simulink model "EV_thermal_charger_2015a_20200311"  (R2015a)
settings: Solver=ode3  StartTime=0.0  StopTime=1800  FixedStep=sampling_time  RelTol=1e-3
PreLoadFcn:
  | run('init_setting.m')
PostLoadFcn:
  | set_param(gcs, 'SimulationCommand', 'update');
  | load('save_param/save_P_Charger', 'P_Charger');
  | load('save_param/save_T_User_set_temp_degC','T_User_set_temp_degC');
  | load('save_param/save_ENV_PNT_PTTH_Temp_add_degC','ENV_PNT_PTTH_Temp_add_degC');
  | load('save_param/save_ENV_PNT_CABIN_Temp_add_degC','ENV_PNT_CABIN_Temp_add_degC');
  | load('save_param/save_ENV_PNT_PHI_Sunlight_W','ENV_PNT_PHI_Sunlight_W');
  | load('save_param/save_ENV_PNT_Outside_Temp_ini_degC','ENV_PNT_Outside_Temp_ini_degC');
undefined symbols (not defined in the file or in its folder): BK_PNT_Pow_UL, BK_PNT_ReGene_vel_limit_DN_kmph, BK_PNT_ReGene_vel_limit_UP_kmph, BK_PNT_Tau_brake, Brk_LL, Brk_PGain, Brk_UL, BT_PNT_Hi_C_pol_hi_batt, BT_PNT_Hi_Capa_hi_batt_F, BT_PNT_Hi_ocv_SOC_hi_batt_OCV_V_table, BT_PNT_Hi_ocv_SOC_hi_batt_OCV_V_table_x_SOC, BT_PNT_Hi_R_hi_batt_cell, BT_PNT_Hi_R_pol_hi_batt, BT_PNT_Hi_SOC_MAX_hi_batt, BT_PNT_Hi_SOC_MIN_hi_batt, BT_PNT_Hi_SOC_START_hi_batt, BT_PNT_Lo_Capa_lo_batt_F, BT_PNT_Lo_ocv_SOC_lo_batt_OCV_V_table, BT_PNT_Lo_ocv_SOC_lo_batt_OCV_V_table_x_SOC, BT_PNT_Lo_R_lo_batt_ohm, BT_PNT_Lo_SOC_MAX_lo_batt, BT_PNT_Lo_SOC_MIN_lo_batt, BT_PNT_Lo_SOC_START_lo_batt, BTTH_CNT_P_BT_Heater_W, BTTH_CNT_P_BT_Heater_W_x_BTCells_degC, BTTH_CNT_Voltage_BTFan_V, BTTH_CNT_Voltage_BTFan_V_x_BTCells_degC, BTTH_PNT_BT_Heat_Resi_KpW, BTTH_PNT_BT_Heat_Resi_KpW_x_Wind_m3ps, BTTH_PNT_BT_Heater2BTCells_Heat_Resi_KpW, BTTH_PNT_BT_Heater_Heat_Capa_JpK, BTTH_PNT_BTBlock2BTAir_Heat_Resi_KpW, BTTH_PNT_BTBlock_Heat_Capa_JpK, BTTH_PNT_BTCells2BTBlock_Heat_Resi_KpW, BTTH_PNT_BTCells_Heat_Capa_JpK, BTTH_PNT_v_BTFan_Wind_vel_mps, BTTH_PNT_v_BTFan_Wind_vel_mps_x_V_BTFan, CATH_CNT_P_Aircon_W_LL, CATH_CNT_P_Aircon_W_UL, CATH_CNT_P_Gain_Aircon, CATH_CNT_P_Gain_PTC_Heater, CATH_CNT_P_Gain_SeatHT, CATH_CNT_P_PTC_Heater, CATH_CNT_P_PTC_Heater_W_LL, CATH_CNT_P_PTC_Heater_W_UL, CATH_CNT_P_PTC_Heater_x_T_Outside_temp_degC, CATH_CNT_P_SeatHT_W_LL, CATH_CNT_P_SeatHT_W_UL, CATH_CNT_PGain_Temp_blowout, CATH_CNT_T_Aircon_Indoor_degC, CATH_CNT_T_Aircon_Indoor_degC_x_T_blowout_degC, CATH_CNT_T_PTC_Heater_degC_UL, CATH_CNT_T_SeatHT_Temp_degC, CATH_CNT_T_SeatHT_Temp_degC_x_T_blowout_degC, CATH_CNT_V_HVAC_Fan, CATH_CNT_V_HVAC_Fan_x_T_blowout_degC, CATH_CNT_V_RDFan_V, CATH_CNT_V_RDFan_x_P_Aircon_W, CATH_PNT_Air_Convection_Heat_Resi_KpW, CATH_PNT_Air_Convection_Heat_Resi_x_mps ... (+141)
undefined symbols (not defined in the file): ACC_D_Gain, ACC_I_Gain, ACC_P_Gain
libraries: METI_Lib_vehicle_model x52, simulink x35
(part 3 of 6)

== system EV_thermal_charger_2015a_20200311/Vehicle/BT_Hi_PNT/Subsystem ==
  I_BT_PNT_A : Inport
  Add : Sum
  Divide : Product
  Resistivity : Constant  Value=BT_PNT_Hi_R_hi_batt_cell
  Transfer Fcn : TransferFcn  Numerator=[BT_PNT_Hi_R_pol_hi_batt]  Denominator=[BT_PNT_Hi_R_pol_hi_batt*BT_PNT_Hi_C_pol_hi_batt 1]
  V_BT_PNT_V : Outport
  wires:
  Resistivity/1 -> Divide/2
  I_BT_PNT_A/1 -> Transfer Fcn/1, Divide/1
  Divide/1 -> Add/1
  Transfer Fcn/1 -> Add/2
  Add/1 -> V_BT_PNT_V/1

== system EV_thermal_charger_2015a_20200311/Vehicle/BT_Lo_PNT/Cal_SOC ==
  I_Lo_BT_PNT_A : Inport
  Capa_batt : Inport  Port=2
  SOC_st : Inport  Port=3
  SOC_MAX : Inport  Port=4
  SOC_MIN : Inport  Port=5
  Clock : Clock
  Memory : Memory
  Memory1 : Memory
  Saturation Dynamic : simulink/Discontinuities/Saturation Dynamic  OutMin=[]  OutMax=[]  OutDataTypeStr=Inherit: Same as second input  OutDataType=fixdt(1, 16)  OutScaling=2^-10  DoSatur=off
  Sum : Sum  Inputs=|++
  Sum1 : Sum  Inputs=++|
  Sum2 : Sum  Inputs=+-|
  Sum5 : Sum  Inputs=|+-
  capa_mn : Product  RndMeth=Zero
  capa_mx : Product  RndMeth=Zero
  capa_mx1 : Product  RndMeth=Zero
  capa_st : Product  RndMeth=Zero
  capa_st1 : Product  Inputs=*/  RndMeth=Zero
  h2sec : Gain  Gain=h2sec
  k : Gain  Gain=percent2mujigen
  k1 : Gain  Gain=percent2mujigen
  k2 : Gain  Gain=percent2mujigen
  k3 : Gain  Gain=mujigen2percent
  SOC_out : Outport
  wires:
  Sum5/1 -> capa_mx1/2
  Memory1/1 -> Sum5/2
  Sum/1 -> Saturation Dynamic/2
  Clock/1 -> Sum5/1, Memory1/1
  capa_mx1/1 -> Sum1/1
  k3/1 -> SOC_out/1
  Sum1/1 -> Sum/2
  Memory/1 -> Sum1/2
  k2/1 -> capa_st/2
  k1/1 -> capa_mn/2
  k/1 -> capa_mx/2
  capa_st/1 -> Sum2/2, Sum/1
  Saturation Dynamic/1 -> Sum2/1, capa_st1/1
  capa_mx/1 -> Saturation Dynamic/1
  capa_mn/1 -> Saturation Dynamic/3
  capa_st1/1 -> k3/1
  h2sec/1 -> capa_mn/1, capa_st1/2, capa_st/1, capa_mx/1
  SOC_MIN/1 -> k1/1
  SOC_MAX/1 -> k/1
  SOC_st/1 -> k2/1
  Capa_batt/1 -> h2sec/1
  I_Lo_BT_PNT_A/1 -> capa_mx1/1
  Sum2/1 -> Memory/1

== system EV_thermal_charger_2015a_20200311/Vehicle/BT_Lo_PNT/Subsystem ==
  I_BT_PNT_Lo_A : Inport
  Divide : Product
  Resistivity : Constant  Value=BT_PNT_Lo_R_lo_batt_ohm
  V_BT_PNT_Lo_V : Outport
  wires:
  Resistivity/1 -> Divide/2
  I_BT_PNT_Lo_A/1 -> Divide/1
  Divide/1 -> V_BT_PNT_Lo_V/1

== system EV_thermal_charger_2015a_20200311/Vehicle/CATH_CNT/Calc_Temp_Blowout ==
  tSetting_T_User_set_temp_degC : Inport
  T_ATM_PNT_Outside_degC : Inport  Port=2
  T_CABA_PNT_T : Inport  Port=3
  v_vehicle_mps_1 : Inport  Port=4
  Add : Sum
  Constant : Constant  Value=CATH_PNT_CABIN_AIR_Heat_Capa_JpK
  Divide : Product  Inputs=*/
  FB : Subsystem
  FF1 : Subsystem
  Gain : Gain  Gain=0.05
  Subtract : Sum  Inputs=-+
  Subtract1 : Sum  Inputs=+-
  T_blowout_degC : Outport
  T_diff_temp_degC : Outport  Port=2
  wires:
  T_CABA_PNT_T/1 -> FF1/2(T_CABIN_AIR_temp_degC), Subtract/2
  T_ATM_PNT_Outside_degC/1 -> FF1/1(T_Outside_temp_degC)
  Add/1 -> Divide/1
  Divide/1 -> Subtract1/2, T_blowout_degC/1
  Constant/1 -> Gain/1
  Subtract/1 -> Subtract1/1, FB/1(T_diff_temp_degC)
  tSetting_T_User_set_temp_degC/1 -> Subtract/1
  Subtract1/1 -> T_diff_temp_degC/1
  FB/1(Q_FB) -> Add/1
  Gain/1 -> Divide/2
  v_vehicle_mps_1/1 -> FF1/3(v_vehicle_mps)
  FF1/1(Q_Heat_Transfar) -> Add/2

== system EV_thermal_charger_2015a_20200311/Vehicle/CATH_CNT/P_Heatpomp_Power_tgt_calc ==
  note: A/CフラグがON かつ Auto Wind ONの時はヒートポンプ稼働
  T_diff_temp_degC : Inport
  T_AC_PNT_Indoor_degC : Inport  Port=2
  Flag_Aircon : Inport  Port=3
  Flag_AutoWind : Inport  Port=4
  Abs : Abs
  Compare To Constant : simulink/Logic and Bit Operations/Compare To Constant  relop=>  const=0.5  OutDataTypeStr=boolean
  Compare To Constant1 : simulink/Logic and Bit Operations/Compare To Constant  relop=>  const=0.5  OutDataTypeStr=boolean
  Constant : Constant  Value=CATH_CNT_P_Gain_Aircon
  Constant1 : Constant  Value=CATH_CNT_P_Aircon_W_UL
  Constant2 : Constant  Value=CATH_CNT_P_Aircon_W_LL
  Constant3 : Constant  Value=0
  Gain1 : Gain  Gain=-1
  Logical Operator : Logic  AllPortsSameDT=off  OutDataTypeStr=boolean
  Product : Product
  Saturation Dynamic : simulink/Discontinuities/Saturation Dynamic  OutMin=[]  OutMax=[]  OutDataTypeStr=Inherit: Same as second input  OutDataType=fixdt(1, 16)  OutScaling=2^-10  DoSatur=off
  Subtract : Sum
  Switch : Switch  Criteria=u2 > Threshold
  T_Aircon_Indoor_tgt : Lookup_n-D  NumberOfTableDimensions=1  BreakpointsForDimension1=CATH_CNT_T_Aircon_Indoor_degC_x_T_blowout_degC  BeginIndexSearchUsingPreviousIndexResult=on  Table=CATH_CNT_T_Aircon_Indoor_degC  ExtrapMethod=Clip  InternalRulePriority=Speed  RndMeth=Simplest  InputSameDT=on
  V_RDFan_tgt1 : Lookup_n-D  NumberOfTableDimensions=1  BreakpointsForDimension1=CATH_CNT_V_RDFan_x_P_Aircon_W  BeginIndexSearchUsingPreviousIndexResult=on  Table=CATH_CNT_V_RDFan_V  ExtrapMethod=Clip  UseLastTableValue=on  InternalRulePriority=Speed  RndMeth=Simplest  InputSameDT=on
  P_CATH_CNT_Heatpomp_W : Outport
  req_V_CATH_CNT_RDFan_V : Outport  Port=2
  wires:
  T_diff_temp_degC/1 -> T_Aircon_Indoor_tgt/1
  T_Aircon_Indoor_tgt/1 -> Subtract/1
  T_AC_PNT_Indoor_degC/1 -> Gain1/1
  Subtract/1 -> Product/1
  Constant/1 -> Product/2
  Product/1 -> Saturation Dynamic/2
  Constant1/1 -> Saturation Dynamic/1
  Constant2/1 -> Saturation Dynamic/3
  Flag_Aircon/1 -> Compare To Constant/1
  Saturation Dynamic/1 -> Switch/1
  Logical Operator/1 -> Switch/2
  Constant3/1 -> Switch/3
  Switch/1 -> Abs/1, P_CATH_CNT_Heatpomp_W/1
  V_RDFan_tgt1/1 -> req_V_CATH_CNT_RDFan_V/1
  Flag_AutoWind/1 -> Compare To Constant1/1
  Compare To Constant/1 -> Logical Operator/1
  Compare To Constant1/1 -> Logical Operator/2
  Gain1/1 -> Subtract/2
  Abs/1 -> V_RDFan_tgt1/1

== system EV_thermal_charger_2015a_20200311/Vehicle/CATH_CNT/P_PTC_Heater_tgt_calc ==
  note: エアコンフラグがONの時は
      | PTCヒーターは使用しない
  note: ヒーター温度が上限値を超過した場合に
      | ヒーター出力を下げる制御
  note: A/CフラグがOFF かつ Auto Wind ONの時
      | PTCヒーターを使用
  T_ATM_PNT_Outside_degC : Inport
  T_PTC_PNT_degC : Inport  Port=2
  Flag_Aircon : Inport  Port=3
  Flag_AutoWind : Inport  Port=4
  Add : Sum
  Compare To Constant : simulink/Logic and Bit Operations/Compare To Constant  relop=>  const=0.5  OutDataTypeStr=boolean
  Compare To Constant1 : simulink/Logic and Bit Operations/Compare To Constant  relop=>  const=0.5  OutDataTypeStr=boolean
  Constant : Constant  Value=CATH_CNT_P_Gain_PTC_Heater
  Constant1 : Constant  Value=CATH_CNT_P_PTC_Heater_W_UL
  Constant2 : Constant  Value=CATH_CNT_P_PTC_Heater_W_LL
  Constant3 : Constant  Value=CATH_CNT_T_PTC_Heater_degC_UL
  Constant4 : Constant  Value=0
  Constant5 : Constant  Value=-inf
  Constant6 : Constant  Value=0
  Logical Operator : Logic  Operator=NOT  AllPortsSameDT=off  OutDataTypeStr=boolean
  Logical Operator1 : Logic  AllPortsSameDT=off  OutDataTypeStr=boolean
  P_PTC_Heater_tgt : Lookup_n-D  NumberOfTableDimensions=1  BreakpointsForDimension1=CATH_CNT_P_PTC_Heater_x_T_Outside_temp_degC  BeginIndexSearchUsingPreviousIndexResult=on  Table=CATH_CNT_P_PTC_Heater  ExtrapMethod=Clip  InternalRulePriority=Speed  RndMeth=Simplest  InputSameDT=on
  Product : Product
  Saturation Dynamic : simulink/Discontinuities/Saturation Dynamic  OutMin=[]  OutMax=[]  OutDataTypeStr=Inherit: Same as second input  OutDataType=fixdt(1, 16)  OutScaling=2^-10  DoSatur=off
  Saturation Dynamic1 : simulink/Discontinuities/Saturation Dynamic  OutMin=[]  OutMax=[]  OutDataTypeStr=Inherit: Same as second input  OutDataType=fixdt(1, 16)  OutScaling=2^-10  DoSatur=off
  Subtract : Sum  Inputs=+-
  Switch : Switch  Criteria=u2 > Threshold
  P_CATH_CNT_PTC_Heater_W : Outport
  wires:
  T_ATM_PNT_Outside_degC/1 -> P_PTC_Heater_tgt/1
  Subtract/1 -> Saturation Dynamic1/2
  Constant/1 -> Product/2
  Add/1 -> Saturation Dynamic/2
  Constant1/1 -> Saturation Dynamic/1
  Constant2/1 -> Saturation Dynamic/3
  T_PTC_PNT_degC/1 -> Subtract/2
  Saturation Dynamic/1 -> Switch/1
  Constant3/1 -> Subtract/1
  Saturation Dynamic1/1 -> Product/1
  Constant4/1 -> Saturation Dynamic1/1
  Constant5/1 -> Saturation Dynamic1/3
  P_PTC_Heater_tgt/1 -> Add/1
  Product/1 -> Add/2
  Flag_Aircon/1 -> Compare To Constant/1
  Compare To Constant/1 -> Logical Operator/1
  Constant6/1 -> Switch/3
  Switch/1 -> P_CATH_CNT_PTC_Heater_W/1
  Logical Operator1/1 -> Switch/2
  Compare To Constant1/1 -> Logical Operator1/2
  Flag_AutoWind/1 -> Compare To Constant1/1
  Logical Operator/1 -> Logical Operator1/1

== system EV_thermal_charger_2015a_20200311/Vehicle/CATH_CNT/Subsystem1 ==
  tSetting_P_Charger : Inport
  Compare To Zero : simulink/Logic and Bit Operations/Compare To Zero  relop=>  OutDataTypeStr=boolean
  Constant1 : Constant
  Constant3 : Constant  Value=0
  Switch : Switch  Criteria=u2 > Threshold
  Switch1 : Switch  Criteria=u2 > Threshold
  Flag_Aircon : Outport
  Flag_AutoWind : Outport  Port=2
  wires:
  Switch/1 -> Flag_Aircon/1
  Switch1/1 -> Flag_AutoWind/1
  Compare To Zero/1 -> Switch1/2, Switch/2
  tSetting_P_Charger/1 -> Compare To Zero/1
  Constant3/1 -> Switch1/1, Switch/1
  Constant1/1 -> Switch1/3, Switch/3

== system EV_thermal_charger_2015a_20200311/Vehicle/CATH_CNT/T_SeatHT_Temp_tgt_calc ==
  T_diff_temp_degC : Inport
  T_SH_PNT_degC : Inport  Port=2
  Constant : Constant  Value=CATH_CNT_P_Gain_SeatHT
  Constant1 : Constant  Value=CATH_CNT_P_SeatHT_W_UL
  Constant2 : Constant  Value=CATH_CNT_P_SeatHT_W_LL
  Product : Product
  Saturation Dynamic : simulink/Discontinuities/Saturation Dynamic  OutMin=[]  OutMax=[]  OutDataTypeStr=Inherit: Same as second input  OutDataType=fixdt(1, 16)  OutScaling=2^-10  DoSatur=off
  Subtract : Sum  Inputs=+-
  T_SeatHT_Temp_tgt : Lookup_n-D  NumberOfTableDimensions=1  BreakpointsForDimension1=CATH_CNT_T_SeatHT_Temp_degC_x_T_blowout_degC  BeginIndexSearchUsingPreviousIndexResult=on  Table=CATH_CNT_T_SeatHT_Temp_degC  ExtrapMethod=Clip  InternalRulePriority=Speed  RndMeth=Simplest  InputSameDT=on
  P_CATH_CNT_SeatHT_W : Outport
  wires:
  T_diff_temp_degC/1 -> T_SeatHT_Temp_tgt/1
  Subtract/1 -> Product/1
  Constant/1 -> Product/2
  Product/1 -> Saturation Dynamic/2
  Constant1/1 -> Saturation Dynamic/1
  Constant2/1 -> Saturation Dynamic/3
  T_SeatHT_Temp_tgt/1 -> Subtract/1
  T_SH_PNT_degC/1 -> Subtract/2
  Saturation Dynamic/1 -> P_CATH_CNT_SeatHT_W/1

== system EV_thermal_charger_2015a_20200311/Vehicle/CATH_CNT/V_HVAC_Fan_calc ==
  T_diff_temp_degC : Inport
  Flag_AutoWind_ON : Inport  Port=2
  Compare To Constant1 : simulink/Logic and Bit Operations/Compare To Constant  relop=>  const=0.5  OutDataTypeStr=boolean
  Constant : Constant  Value=0
  Switch : Switch  Criteria=u2 > Threshold  Threshold=0.5
  V_HVAC_Fan : Lookup_n-D  NumberOfTableDimensions=1  BreakpointsForDimension1=CATH_CNT_V_HVAC_Fan_x_T_blowout_degC  BeginIndexSearchUsingPreviousIndexResult=on  Table=CATH_CNT_V_HVAC_Fan  ExtrapMethod=Clip  InternalRulePriority=Speed  RndMeth=Simplest  InputSameDT=on
  V_CATH_CNT_Aircon_Fan_V : Outport
  wires:
  T_diff_temp_degC/1 -> V_HVAC_Fan/1
  V_HVAC_Fan/1 -> Switch/1
  Flag_AutoWind_ON/1 -> Compare To Constant1/1
  Constant/1 -> Switch/3
  Switch/1 -> V_CATH_CNT_Aircon_Fan_V/1
  Compare To Constant1/1 -> Switch/2

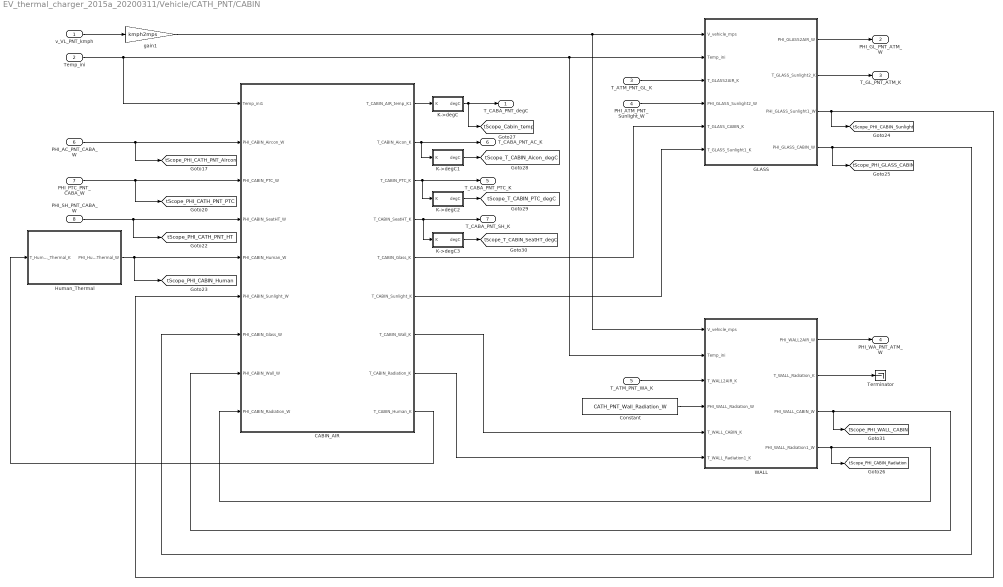
== system EV_thermal_charger_2015a_20200311/Vehicle/CATH_PNT/CABIN ==
  v_VL_PNT_kmph : Inport
  Temp_ini : Inport  Port=2
  T_ATM_PNT_GL_K : Inport  Port=3
  PHI_ATM_PNT_Sunlight_W : Inport  Port=4
  T_ATM_PNT_WA_K : Inport  Port=5
  PHI_AC_PNT_CABA_W : Inport  Port=6
  PHI_PTC_PNT_CABA_W : Inport  Port=7
  PHI_SH_PNT_CABA_W : Inport  Port=8
  CABIN_AIR : Subsystem
  Constant : Constant  Value=CATH_PNT_Wall_Radiation_W
  GLASS : Subsystem
  Human_Thermal : Subsystem
  K->degC : Subsystem
  K->degC1 : Subsystem
  K->degC2 : Subsystem
  K->degC3 : Subsystem
  Terminator : Terminator
  WALL : Subsystem
  gain1 : Gain  Gain=kmph2mps
  T_CABA_PNT_degC : Outport
  PHI_GL_PNT_ATM_W : Outport  Port=2
  T_GL_PNT_ATM_K : Outport  Port=3
  PHI_WA_PNT_ATM_W : Outport  Port=4
  T_CABA_PNT_PTC_K : Outport  Port=5
  T_CABA_PNT_AC_K : Outport  Port=6
  T_CABA_PNT_SH_K : Outport  Port=7
  tag scope: tScope_Cabin_temp=global, tScope_PHI_CABIN_Human=global, tScope_PHI_CABIN_Radiation=global, tScope_PHI_CABIN_Sunlight=global, tScope_PHI_CATH_PNT_Aircon=global, tScope_PHI_CATH_PNT_HT=global, tScope_PHI_CATH_PNT_PTC=global, tScope_PHI_GLASS_CABIN=global, tScope_PHI_WALL_CABIN=global, tScope_T_CABIN_Aicon_degC=global, tScope_T_CABIN_PTC_degC=global, tScope_T_CABIN_SeatHT_degC=global
  wires:
  CABIN_AIR/6(T_CABIN_Sunlight_K) -> GLASS/6(T_GLASS_Sunlight1_K)
  T_ATM_PNT_GL_K/1 -> GLASS/3(T_GLASS2AIR_K)
  GLASS/1(PHI_GLASS2AIR_W) -> PHI_GL_PNT_ATM_W/1
  CABIN_AIR/8(T_CABIN_Radiation_K) -> WALL/6(T_WALL_Radiation1_K)
  WALL/1(PHI_WALL2AIR_W) -> PHI_WA_PNT_ATM_W/1
  T_ATM_PNT_WA_K/1 -> WALL/3(T_WALL2AIR_K)
  CABIN_AIR/9(T_CABIN_Human_K) -> Human_Thermal/1(T_Human_Thermal_K)
  GLASS/2(T_GLASS_Sunlight2_K) -> T_GL_PNT_ATM_K/1
  PHI_ATM_PNT_Sunlight_W/1 -> GLASS/4(PHI_GLASS_Sunlight2_W)
  CABIN_AIR/1(T_CABIN_AIR_temp_K1) -> K->degC/1(K)
  K->degC/1(degC) -> T_CABA_PNT_degC/1, [tScope_Cabin_temp]
  Temp_ini/1 -> GLASS/2(Temp_ini), WALL/2(Temp_ini), CABIN_AIR/1(Temp_ini1)
  CABIN_AIR/5(T_CABIN_Glass_K) -> GLASS/5(T_GLASS_CABIN_K)
  CABIN_AIR/7(T_CABIN_Wall_K) -> WALL/5(T_WALL_CABIN_K)
  v_VL_PNT_kmph/1 -> gain1/1
  Constant/1 -> WALL/4(PHI_WALL_Radiation_W)
  WALL/2(T_WALL_Radiation_K) -> Terminator/1
  gain1/1 -> GLASS/1(V_vehicle_mps), WALL/1(V_vehicle_mps)
  Human_Thermal/1(PHI_Human_Thermal_W) -> [tScope_PHI_CABIN_Human], CABIN_AIR/5(PHI_CABIN_Human_W)
  K->degC1/1(degC) -> [tScope_T_CABIN_Aicon_degC]
  K->degC2/1(degC) -> [tScope_T_CABIN_PTC_degC]
  K->degC3/1(degC) -> [tScope_T_CABIN_SeatHT_degC]
  PHI_AC_PNT_CABA_W/1 -> CABIN_AIR/2(PHI_CABIN_Aircon_W), [tScope_PHI_CATH_PNT_Aircon]
  PHI_PTC_PNT_CABA_W/1 -> [tScope_PHI_CATH_PNT_PTC], CABIN_AIR/3(PHI_CABIN_PTC_W)
  PHI_SH_PNT_CABA_W/1 -> [tScope_PHI_CATH_PNT_HT], CABIN_AIR/4(PHI_CABIN_SeatHT_W)
  CABIN_AIR/2(T_CABIN_Aicon_K) -> T_CABA_PNT_AC_K/1, K->degC1/1(K)
  CABIN_AIR/3(T_CABIN_PTC_K) -> T_CABA_PNT_PTC_K/1, K->degC2/1(K)
  CABIN_AIR/4(T_CABIN_SeatHT_K) -> T_CABA_PNT_SH_K/1, K->degC3/1(K)
  GLASS/3(PHI_GLASS_Sunlight1_W) -> CABIN_AIR/6(PHI_CABIN_Sunlight_W), [tScope_PHI_CABIN_Sunlight]
  WALL/4(PHI_WALL_Radiation1_W) -> [tScope_PHI_CABIN_Radiation], CABIN_AIR/9(PHI_CABIN_Radiation_W)
  GLASS/4(PHI_GLASS_CABIN_W) -> [tScope_PHI_GLASS_CABIN], CABIN_AIR/7(PHI_CABIN_Glass_W)
  WALL/3(PHI_WALL_CABIN_W) -> [tScope_PHI_WALL_CABIN], CABIN_AIR/8(PHI_CABIN_Wall_W)

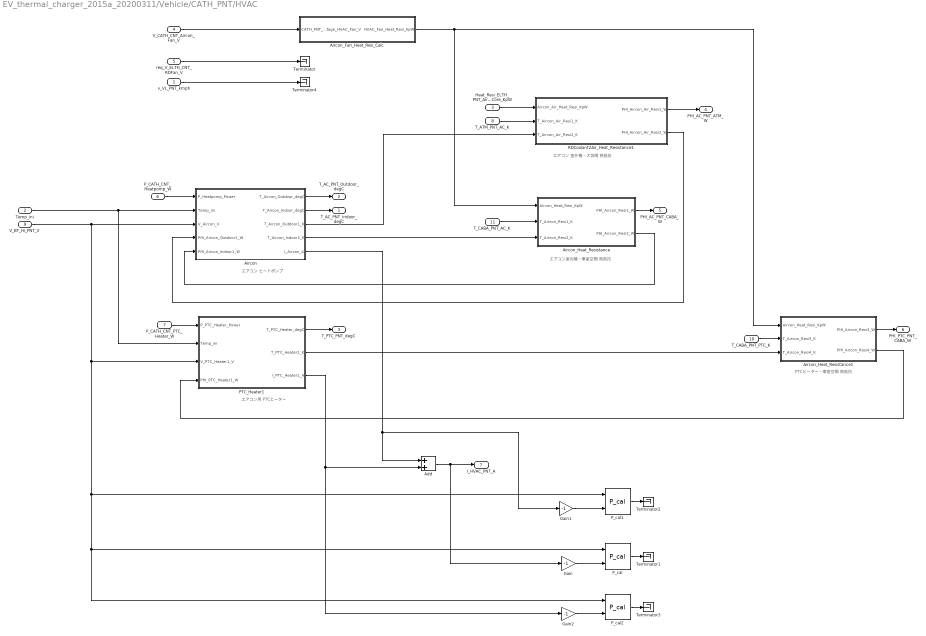
== system EV_thermal_charger_2015a_20200311/Vehicle/CATH_PNT/HVAC ==
  note: エアコン用
      | PTCヒーター
  note: エアコン
      | ヒートポンプ
  note: エアコン 室外機～大気間
      | 熱抵抗
  note: エアコン室内機～車室空間
      | 熱抵抗
  note: PTCヒーター～車室空間
      | 熱抵抗
  v_VL_PNT_kmph : Inport
  Temp_ini : Inport  Port=2
  Heat_Resi_ELTH_PNT_AirconCore_KpW : Inport  Port=3
  V_CATH_CNT_Aircon_Fan_V : Inport  Port=4
  req_V_ELTH_CNT_RDFan_V : Inport  Port=5
  P_CATH_CNT_Heatpomp_W : Inport  Port=6
  P_CATH_CNT_PTC_Heater_W : Inport  Port=7
  T_ATM_PNT_AC_K : Inport  Port=8
  V_BT_Hi_PNT_V : Inport  Port=9
  T_CABA_PNT_PTC_K : Inport  Port=10
  T_CABA_PNT_AC_K : Inport  Port=11
  Add : Sum
  Aircon : Subsystem
  Aircon_Fan_Heat_Resi_Calc : Subsystem
  Aircon_Heat_Resistance : Subsystem
  Aircon_Heat_Resistance1 : Subsystem
  Gain : Gain  Gain=-1
  Gain1 : Gain  Gain=-1
  Gain2 : Gain  Gain=-1
  PTC_Heater1 : Subsystem
  P_cal : METI_Lib_vehicle_model/P_cal  Type_energy=電気  Type_output_energy=損失  Power_name=Pl_  t_Workspace_Name=EL_HVAC  P_VariableName=Pl_EL_HVAC  Across_VariableName=V_EL_HVAC  Throgh_VariableName=I_EL_HVAC
  P_cal1 : METI_Lib_vehicle_model/P_cal  Type_energy=電気  Type_output_energy=損失  Power_name=Pl_  t_Workspace_Name=EL_Aircon_Comp  P_VariableName=Pl_EL_Aircon_Comp  Across_VariableName=V_EL_Aircon_Comp  Throgh_VariableName=I_EL_Aircon_Comp
  P_cal2 : METI_Lib_vehicle_model/P_cal  Type_energy=電気  Type_output_energy=損失  Power_name=Pl_  t_Workspace_Name=EL_HVAC_PTC  P_VariableName=Pl_EL_HVAC_PTC  Across_VariableName=V_EL_HVAC_PTC  Throgh_VariableName=I_EL_HVAC_PTC
  RDCoolant2Air_Heat_Resistance1 : Subsystem
  Terminator{,1..4} (5 alike) : Terminator
  T_AC_PNT_Indoor_degC : Outport
  T_AC_PNT_Outdoor_degC : Outport  Port=2
  T_PTC_PNT_degC : Outport  Port=3
  PHI_AC_PNT_ATM_W : Outport  Port=4
  PHI_AC_PNT_CABA_W : Outport  Port=5
  PHI_PTC_PNT_CABA_W : Outport  Port=6
  I_HVAC_PNT_A : Outport  Port=7
  wires:
  T_ATM_PNT_AC_K/1 -> RDCoolant2Air_Heat_Resistance1/2(T_Aircon_Air_Resi1_K)
  T_CABA_PNT_AC_K/1 -> Aircon_Heat_Resistance/2(T_Aircon_Resi1_K)
  Add/1 -> I_HVAC_PNT_A/1, Gain/1
  RDCoolant2Air_Heat_Resistance1/1(PHI_Aircon_Air_Resi1_W) -> PHI_AC_PNT_ATM_W/1
  Aircon_Heat_Resistance/1(PHI_Aircon_Resi1_W) -> PHI_AC_PNT_CABA_W/1
  Aircon_Heat_Resistance1/1(PHI_Aircon_Resi3_W) -> PHI_PTC_PNT_CABA_W/1
  T_CABA_PNT_PTC_K/1 -> Aircon_Heat_Resistance1/2(T_Aircon_Resi3_K)
  Aircon/3(T_Aircon_Outdoor1_K) -> RDCoolant2Air_Heat_Resistance1/3(T_Aircon_Air_Resi2_K)
  req_V_ELTH_CNT_RDFan_V/1 -> Terminator/1
  Heat_Resi_ELTH_PNT_AirconCore_KpW/1 -> RDCoolant2Air_Heat_Resistance1/1("Aircon_Air_Heat_Resi_KpW ")
  RDCoolant2Air_Heat_Resistance1/2(PHI_Aircon_Air_Resi2_W) -> Aircon/4(PHI_Aircon_Outdoor1_W)
  v_VL_PNT_kmph/1 -> Terminator4/1
  Aircon_Heat_Resistance/2(PHI_Aircon_Resi2_W) -> Aircon/5(PHI_Aircon_Indoor1_W)
  P_CATH_CNT_PTC_Heater_W/1 -> PTC_Heater1/1(P_PTC_Heater_Power)
  PTC_Heater1/3(I_PTC_Heater1_A) -> Gain2/1, Add/2
  P_CATH_CNT_Heatpomp_W/1 -> Aircon/1(P_Heatpomp_Power)
  Temp_ini/1 -> Aircon/2(Temp_ini), PTC_Heater1/2(Temp_ini)
  Aircon/5(I_Aircon_A) -> Gain1/1, Add/1
  Aircon_Fan_Heat_Resi_Calc/1("HVAC_Fan_Heat_Resi_KpW ") -> Aircon_Heat_Resistance/1("Aircon_Heat_Resi_KpW "), Aircon_Heat_Resistance1/1("Aircon_Heat_Resi_KpW ")
  V_CATH_CNT_Aircon_Fan_V/1 -> Aircon_Fan_Heat_Resi_Calc/1(CATH_PNT_Voltage_HVAC_Fan_V)
  Aircon/2(T_Aircon_Indoor_degC) -> T_AC_PNT_Indoor_degC/1
  PTC_Heater1/1(T_PTC_Heater_degC) -> T_PTC_PNT_degC/1
  PTC_Heater1/2(T_PTC_Heater1_K) -> Aircon_Heat_Resistance1/3(T_Aircon_Resi4_K)
  Aircon_Heat_Resistance1/2(PHI_Aircon_Resi4_W) -> PTC_Heater1/4(PHI_PTC_Heater1_W)
  Aircon/4(T_Aircon_Indoor1_K) -> Aircon_Heat_Resistance/3(T_Aircon_Resi2_K)
  Aircon/1(T_Aircon_Outdoor_degC) -> T_AC_PNT_Outdoor_degC/1
  P_cal/1 -> Terminator1/1
  Gain/1 -> P_cal/2
  P_cal1/1 -> Terminator2/1
  Gain1/1 -> P_cal1/2
  P_cal2/1 -> Terminator3/1
  V_BT_Hi_PNT_V/1 -> P_cal2/1, P_cal/1, P_cal1/1, PTC_Heater1/3(V_PTC_Heater1_V), Aircon/3(V_Aircon_V)
  Gain2/1 -> P_cal2/2

== system EV_thermal_charger_2015a_20200311/Vehicle/CATH_PNT/Seat_Heater ==
  Temp_ini : Inport
  P_CATH_CNT_SeatHT_W : Inport  Port=2
  V_BT_Lo_PNT_V : Inport  Port=3
  T_CABA_PNT_SH_K : Inport  Port=4
  Gain : Gain  Gain=-1
  K->degC : Subsystem
  P_cal : METI_Lib_vehicle_model/P_cal  Type_energy=電気  Type_output_energy=損失  Power_name=Pl_  t_Workspace_Name=EL_Seat_Heater  P_VariableName=Pl_EL_Seat_Heater  Across_VariableName=V_EL_Seat_Heater  Throgh_VariableName=I_EL_Seat_Heater
  SeatHT_Heat_Capacity : Subsystem
  Seat_HT : Subsystem
  Seat_Heater_Heat_Resistance : Subsystem
  Terminator1 : Terminator
  PHI_SH_PNT_CABA_W : Outport
  T_SeatHT_Temp_degC : Outport  Port=2
  T_SH_PNT_degC : Outport  Port=3
  wires:
  SeatHT_Heat_Capacity/2(T_SeatHT1_K) -> Seat_HT/3(T_Seat_HT_K)
  Seat_Heater_Heat_Resistance/2(PHI_SeatHT_Resi2_W) -> SeatHT_Heat_Capacity/3(PHI_SeatHT2_W)
  SeatHT_Heat_Capacity/1(T_SeatHT2_K) -> Seat_Heater_Heat_Resistance/1(T_SeatHT_Resi2_K), K->degC/1(K)
  Temp_ini/1 -> SeatHT_Heat_Capacity/1(Temp_ini)
  T_CABA_PNT_SH_K/1 -> Seat_Heater_Heat_Resistance/2(T_SeatHT_Resi1_K)
  Seat_Heater_Heat_Resistance/1(PHI_SeatHT_Resi1_W) -> PHI_SH_PNT_CABA_W/1
  K->degC/1(degC) -> T_SeatHT_Temp_degC/1
  P_CATH_CNT_SeatHT_W/1 -> Seat_HT/1(P_Seat_Heater_Power)
  Seat_HT/2(I_Seat_HT_A) -> T_SH_PNT_degC/1, Gain/1
  P_cal/1 -> Terminator1/1
  Gain/1 -> P_cal/2
  V_BT_Lo_PNT_V/1 -> Seat_HT/2(V_Seat_HT_V), P_cal/1
  Seat_HT/1(PHI_Seat_HT_W) -> SeatHT_Heat_Capacity/2(PHI_SeatHT1_W)

== system EV_thermal_charger_2015a_20200311/Vehicle/CHG_CNT/Charge_Current_calc ==
  note: 0：接続ネゴシエーション
      | 1：初期充電
      | 2：本充電
  Charge_mode : Inport
  V_CHG_PNT_Charge_V : Inport  Port=2
  SOC_BT_Hi_PNT_per : Inport  Port=3
  Maximum_Hi_Batt_SOC : Inport  Port=4
  Constant : Constant  Value=P_Charger
  Constant4 : Constant  Value=CHG_CNT_Initial_Charge_Current_A
  Constant5 : Constant  Value=CHG_CNT_Maximum_Charge_Current_A
  Constant6 : Constant  Value=CHG_CNT_Maximum_Charge_Power_W
  Constant7 : Constant  Value=CHG_CNT_Maximum_Charge_Voltage_V
  If : If  IfExpression=u1 < 0.5  ElseIfExpressions=u1 < 1.5
  Initial_Charge : Subsystem  TreatAsAtomicUnit=on
  Manual Switch : ManualSwitch
  Merge : Merge  Inputs=3
  Negotiation_time : Subsystem  TreatAsAtomicUnit=on
  Normal_Charge : Subsystem  TreatAsAtomicUnit=on
  Current_tgt : Outport
  wires:
  Manual Switch/1 -> Normal_Charge/2(Maximum_Charge_Power_W)
  Constant7/1 -> Normal_Charge/3(Maximum_Charge_Voltage_V)
  Negotiation_time/1(Out1) -> Merge/1
  Constant4/1 -> Initial_Charge/1(In1)
  Charge_mode/1 -> If/1
  Constant5/1 -> Normal_Charge/1(Maximum_Charge_Current_A)
  If/2 -> Initial_Charge/Action
  If/1 -> Negotiation_time/Action
  Initial_Charge/1(Out1) -> Merge/2
  If/3 -> Normal_Charge/Action
  Merge/1 -> Current_tgt/1
  Normal_Charge/1(Current_tgt) -> Merge/3
  V_CHG_PNT_Charge_V/1 -> Normal_Charge/4(Battery_Voltage_V)
  SOC_BT_Hi_PNT_per/1 -> Normal_Charge/5(SOC_HiBatt)
  Maximum_Hi_Batt_SOC/1 -> Normal_Charge/6(Maximum_Hi_Batt_SOC)
  Constant/1 -> Manual Switch/2
  Constant6/1 -> Manual Switch/1

== system EV_thermal_charger_2015a_20200311/Vehicle/CHG_CNT/Current_rate_limitter ==
  Current_tgt_In1 : Inport
  SOC_BT_Hi_PNT_per : Inport  Port=2
  SOC_UL : Inport  Port=3
  Compare To Zero : simulink/Logic and Bit Operations/Compare To Zero  relop=<  OutDataTypeStr=boolean
  Constant10 : Constant  Value=CHG_CNT_charge_current_rate_UL
  Constant11 : Constant  Value=CHG_CNT_charge_current_rate_LL
  Constant9 : Constant  Value=0
  Rate Limiter Dynamic : simulink/Discontinuities/Rate Limiter Dynamic
  Subtract : Sum  Inputs=+-
  Switch : Switch  Criteria=u2 > Threshold
  tgt_I_CHG_CNT_Charge_A : Outport
  wires:
  Constant11/1 -> Rate Limiter Dynamic/3
  Constant9/1 -> Switch/3
  Rate Limiter Dynamic/1 -> tgt_I_CHG_CNT_Charge_A/1
  Subtract/1 -> Compare To Zero/1
  Switch/1 -> Rate Limiter Dynamic/2
  Compare To Zero/1 -> Switch/2
  Constant10/1 -> Rate Limiter Dynamic/1
  SOC_UL/1 -> Subtract/2
  SOC_BT_Hi_PNT_per/1 -> Subtract/1
  Current_tgt_In1/1 -> Switch/1

== system EV_thermal_charger_2015a_20200311/Vehicle/CHG_CNT/counter ==
  note: カウントした数値＞設定数値となったら
      | 1を出力
  note: signal=1でカウントスタート
      | time stepの数字を毎ステップ加算していく
      | signal=0でリセット
  signal : Inport
  time_step : Inport  Port=2
  count_time : Inport  Port=3
  Add : Sum
  Constant : Constant  Value=0
  Constant1 : Constant  Value=0
  Constant2 : Constant
  Memory : Memory
  Product : Product
  Subtract : Sum  Inputs=+-
  Switch : Switch  Criteria=u2 > Threshold  Threshold=0.5
  Switch1 : Switch  Criteria=u2 > Threshold
  Out1 : Outport
  wires:
  signal/1 -> Product/1, Switch/2
  Product/1 -> Add/1
  time_step/1 -> Product/2
  Constant/1 -> Switch/3
  Memory/1 -> Switch/1
  Add/1 -> Memory/1, Subtract/1
  Switch/1 -> Add/2
  count_time/1 -> Subtract/2
  Subtract/1 -> Switch1/2
  Switch1/1 -> Out1/1
  Constant1/1 -> Switch1/3
  Constant2/1 -> Switch1/1

== system EV_thermal_charger_2015a_20200311/Vehicle/CHG_CNT/counter1 ==
  note: カウントした数値＞設定数値となったら
      | 1を出力
  note: signal=1でカウントスタート
      | time stepの数字を毎ステップ加算していく
      | signal=0でリセット
  signal : Inport
  time_step : Inport  Port=2
  count_time : Inport  Port=3
  Add : Sum
  Constant : Constant  Value=0
  Constant1 : Constant  Value=0
  Constant2 : Constant
  Memory : Memory
  Product : Product
  Subtract : Sum  Inputs=+-
  Switch : Switch  Criteria=u2 > Threshold  Threshold=0.5
  Switch1 : Switch  Criteria=u2 > Threshold
  Out1 : Outport
  wires:
  signal/1 -> Product/1, Switch/2
  Product/1 -> Add/1
  time_step/1 -> Product/2
  Constant/1 -> Switch/3
  Memory/1 -> Switch/1
  Add/1 -> Memory/1, Subtract/1
  Switch/1 -> Add/2
  count_time/1 -> Subtract/2
  Subtract/1 -> Switch1/2
  Switch1/1 -> Out1/1
  Constant1/1 -> Switch1/3
  Constant2/1 -> Switch1/1

== system EV_thermal_charger_2015a_20200311/Vehicle/DCDC_PNT/Controller ==
  note: 0割防止
  Target V : Inport
  V : Inport  Port=2
  Constant : Constant  Value=0.01
  Divide : Product  Inputs=*/
  MinMax : MinMax  Function=max  Inputs=2
  Gain : Outport
  wires:
  Divide/1 -> Gain/1
  Target V/1 -> Divide/1
  MinMax/1 -> Divide/2
  V/1 -> MinMax/1
  Constant/1 -> MinMax/2

== system EV_thermal_charger_2015a_20200311/Vehicle/DCDC_PNT/resi1 ==
  In1 : Inport
  Constant1 : Constant  Value=DCDC_PNT_R_conv_lo
  Product4 : Product  Inputs=*/  RndMeth=Zero
  Out1 : Outport
  wires:
  In1/1 -> Product4/1
  Constant1/1 -> Product4/2
  Product4/1 -> Out1/1

== system EV_thermal_charger_2015a_20200311/Vehicle/DF_PNT/DriveShaft ==
  "w_DF_PNT_radps " : Inport
  "w_TR_PNT_radps " : Inport  Port=2
  Add : Sum  Inputs=+-
  Add1 : Sum
  Discrete-Time Integrator : DiscreteIntegrator  InitialConditionSetting=State (most efficient)  SampleTime=sampling_time  LowerSaturationLimit=0
  Gain : Gain  Gain=-1
  Gain1 : Gain  Gain=DF_PNT_Driveshaft_spring
  Gain2 : Gain  Gain=DF_PNT_Driveshaft_damper
  "Trq_DF_PNT_Nm " : Outport
  Trq_DF_PNT_DN_Nm : Outport  Port=2
  wires:
  Discrete-Time Integrator/1 -> Gain1/1
  "w_DF_PNT_radps "/1 -> Add/1
  "w_TR_PNT_radps "/1 -> Add/2
  Gain1/1 -> Add1/1
  Gain2/1 -> Add1/2
  Gain/1 -> "Trq_DF_PNT_Nm "/1
  Add/1 -> Discrete-Time Integrator/1, Gain2/1
  Add1/1 -> Trq_DF_PNT_DN_Nm/1, Gain/1

== system EV_thermal_charger_2015a_20200311/Vehicle/ELTH_PNT/INVTH_PNT ==
  note: モーターハウジングへの熱量
  note: ヒートシンクの
      | 熱容量
  note: インバータ筐体の
      | 熱容量
  note: 冷却水からの熱量
  Temp_ini : Inport
  PHI_INV_PNT_W : Inport  Port=2
  T_ATM_PNT_INV_K : Inport  Port=3
  T_MGTH_PNT_INVTH_K : Inport  Port=4
  PHI_RD_PNT_INVTH_W : Inport  Port=5
  INVBlock2Air_Heat_Resistance : Subsystem
  INVBlock_Heat_Capacity : Subsystem
  INVHeatsink2INVBlock_Heat_Resistance : Subsystem
  INVTH_Heatsink_Heat_Capacity : Subsystem
  K->degC1 : Subsystem
  K->degC2 : Subsystem
  MG2INVBlock_Heat_Resistance : Subsystem
  T_INVHeatsink_K : Outport
  T_INVTH_PNT_K : Outport  Port=2
  PHI_INVTH_PNT_ATM_W : Outport  Port=3
  T_INVTH_PNT_RD_K : Outport  Port=4
  PHI_INVTH_PNT_MGTH_W : Outport  Port=5
  tag scope: tScope_T_INVBlock_degC=global, tScope_T_INVHeatsink_degC=global
  wires:
  INVBlock_Heat_Capacity/3(T_INVBlock1_K) -> INVHeatsink2INVBlock_Heat_Resistance/2(T_INVBlock_Resi1_K)
  INVHeatsink2INVBlock_Heat_Resistance/1(PHI_INVBlock_Resi1_W) -> INVBlock_Heat_Capacity/3(PHI_INVBlock1_W)
  INVBlock2Air_Heat_Resistance/2(PHI_INVBlock_Resi3_W) -> INVBlock_Heat_Capacity/4(PHI_INVBlock3_W)
  INVBlock_Heat_Capacity/2(T_INVBlock3_K) -> INVBlock2Air_Heat_Resistance/2(T_INVBlock_Resi3_K), K->degC1/1(K)
  INVBlock2Air_Heat_Resistance/1(PHI_INV2Air_Resi1_W) -> PHI_INVTH_PNT_ATM_W/1
  MG2INVBlock_Heat_Resistance/1(PHI_INVBlock_Resi2_W) -> INVBlock_Heat_Capacity/1(PHI_INVBlock2_W)
  INVBlock_Heat_Capacity/1(T_INVBlock2_K) -> MG2INVBlock_Heat_Resistance/1(T_INVBlock_Resi2_K)
  T_MGTH_PNT_INVTH_K/1 -> MG2INVBlock_Heat_Resistance/2(T_MGBlock_Resi4_K)
  MG2INVBlock_Heat_Resistance/2(PHI_MGBlock_Resi4_W) -> PHI_INVTH_PNT_MGTH_W/1
  INVTH_Heatsink_Heat_Capacity/1(T_INVTH_Heatsink1_K) -> T_INVTH_PNT_K/1
  PHI_INV_PNT_W/1 -> INVTH_Heatsink_Heat_Capacity/2(PHI_INVTH_Heatsink1_W)
  T_ATM_PNT_INV_K/1 -> INVBlock2Air_Heat_Resistance/1(T_INV2Air_Resi1_K)
  INVTH_Heatsink_Heat_Capacity/3(T_INVTH_Heatsink3_K) -> T_INVTH_PNT_RD_K/1, K->degC2/1(K), T_INVHeatsink_K/1  "T_INVHeatsink_K"
  PHI_RD_PNT_INVTH_W/1 -> INVTH_Heatsink_Heat_Capacity/3(PHI_INVTH_Heatsink3_W)
  INVTH_Heatsink_Heat_Capacity/2(T_INVTH_Heatsink2_K) -> INVHeatsink2INVBlock_Heat_Resistance/1(T_INVHeatsink_Resi2_K)
  INVHeatsink2INVBlock_Heat_Resistance/2(PHI_INVHeatsink_Resi2_W) -> INVTH_Heatsink_Heat_Capacity/4(PHI_INVTH_Heatsink2_W)
  Temp_ini/1 -> INVTH_Heatsink_Heat_Capacity/1(Temp_ini), INVBlock_Heat_Capacity/2(Temp_ini)
  K->degC2/1(degC) -> [tScope_T_INVHeatsink_degC]
  K->degC1/1(degC) -> [tScope_T_INVBlock_degC]

== system EV_thermal_charger_2015a_20200311/Vehicle/ELTH_PNT/K->degC1 ==
  K : Inport
  Constant2 : Constant  Value=K2degC
  Sum : Sum  Inputs=++|
  degC : Outport
  wires:
  K/1 -> Sum/2
  Constant2/1 -> Sum/1
  Sum/1 -> degC/1

== system EV_thermal_charger_2015a_20200311/Vehicle/ELTH_PNT/K->degC3 ==
  K : Inport
  Constant2 : Constant  Value=K2degC
  Sum : Sum  Inputs=++|
  degC : Outport
  wires:
  K/1 -> Sum/2
  Constant2/1 -> Sum/1
  Sum/1 -> degC/1

== system EV_thermal_charger_2015a_20200311/Vehicle/ELTH_PNT/K->degC6 ==
  K : Inport
  Constant2 : Constant  Value=K2degC
  Sum : Sum  Inputs=++|
  degC : Outport
  wires:
  K/1 -> Sum/2
  Constant2/1 -> Sum/1
  Sum/1 -> degC/1

== system EV_thermal_charger_2015a_20200311/Vehicle/ELTH_PNT/MGTH_PNT ==
  note: モーターコイルの
      | 熱容量
  note: モーターハウジングの
      | 熱容量
  note: インバータ筐体からの熱量
  note: PTサーマルシステムへの熱量
  note: 冷却水から
      | モーターハウジングへの熱量
  note: モーターの損失が
      | コイルへの熱量
  note: モーターハウジングから大気へ
      | 放熱する熱量
  Temp_ini : Inport
  PHI_MG_PNT_W : Inport  Port=2
  T_TMTH_PNT_ELTH_K : Inport  Port=3
  T_ATM_PNT_MG_K : Inport  Port=4
  " PHI_RD_PNT_MGTH_W" : Inport  Port=5
  PHI_INVTH_PNT_MGTH_W : Inport  Port=6
  Coil_Heat_Capacity : Subsystem
  K->degC1 : Subsystem
  K->degC2 : Subsystem
  MGCoil2MGHousing_Heat_Resistance : Subsystem
  MGHousing2Air_Heat_Resistance : Subsystem
  MGHousing_Heat_Capacity : Subsystem
  PTTH2MGHousing_Heat_Resistance : Subsystem
  T_MGCoil_K : Outport
  T_MGTH_PNT_K : Outport  Port=2
  PHI_MGTH_PNT_PTTH_W : Outport  Port=3
  PHI_MGTH_PNT_ATM_W : Outport  Port=4
  T_MGTH_PNT_RD_K : Outport  Port=5
  T_MGTH_PNT_INVTH_K : Outport  Port=6
  tag scope: tScope_T_MGBlock_degC=global, tScope_T_MGCoil_degC=global
  wires:
  Coil_Heat_Capacity/2(T_MGCoil2_K) -> MGCoil2MGHousing_Heat_Resistance/1(T_MGCoil_Resi4_K), K->degC1/1(K)
  MGCoil2MGHousing_Heat_Resistance/2(PHI_MGCoil_Resi4_W) -> Coil_Heat_Capacity/3(PHI_MGCoil2_W)
  MGHousing_Heat_Capacity/5(T_MGHousing1_K) -> MGCoil2MGHousing_Heat_Resistance/2(T_MGHousing_Resi1_K)
  Coil_Heat_Capacity/1(T_MGCoil1_K) -> T_MGTH_PNT_K/1, T_MGCoil_K/1  "T_MGCoil_K"
  PHI_MG_PNT_W/1 -> Coil_Heat_Capacity/2(PHI_MGCoil1_W)
  T_TMTH_PNT_ELTH_K/1 -> PTTH2MGHousing_Heat_Resistance/2(T_PTTH_Resi2_K)
  PTTH2MGHousing_Heat_Resistance/2(PHI_PTTH_Resi2_W) -> PHI_MGTH_PNT_PTTH_W/1
  PTTH2MGHousing_Heat_Resistance/1(PHI_MGHousing_Resi2_W) -> MGHousing_Heat_Capacity/1(PHI_MGHousing2_W)
  MGHousing_Heat_Capacity/1(T_MGHousing2_K) -> PTTH2MGHousing_Heat_Resistance/1(T_MGHousing_Resi2_K)
  T_ATM_PNT_MG_K/1 -> MGHousing2Air_Heat_Resistance/1(T_MG2Air_Resi1_K)
  MGHousing2Air_Heat_Resistance/1(PHI_MG2Air_Resi1_W) -> PHI_MGTH_PNT_ATM_W/1
  MGHousing_Heat_Capacity/3(T_MGHousing4_K) -> T_MGTH_PNT_INVTH_K/1
  PHI_INVTH_PNT_MGTH_W/1 -> MGHousing_Heat_Capacity/3(PHI_MGHousing4_W)
  MGHousing_Heat_Capacity/4(T_MGHousing5_K) -> K->degC2/1(K), MGHousing2Air_Heat_Resistance/2(T_MGHousing_Resi5_K)
  MGHousing2Air_Heat_Resistance/2(PHI_MGHousing_Resi5_W) -> MGHousing_Heat_Capacity/6(PHI_MGHousing5_W)
  MGHousing_Heat_Capacity/2(T_MGHousing3_K) -> T_MGTH_PNT_RD_K/1
  " PHI_RD_PNT_MGTH_W"/1 -> MGHousing_Heat_Capacity/2(PHI_MGHousing3_W)
  Temp_ini/1 -> Coil_Heat_Capacity/1(Temp_ini), MGHousing_Heat_Capacity/4(Temp_ini)
  K->degC1/1(degC) -> [tScope_T_MGCoil_degC]
  K->degC2/1(degC) -> [tScope_T_MGBlock_degC]
  MGCoil2MGHousing_Heat_Resistance/1(PHI_MGHousing_Resi1_W) -> MGHousing_Heat_Capacity/5(PHI_MGHousing1_W)

== system EV_thermal_charger_2015a_20200311/Vehicle/ELTH_PNT/RD_PNT ==
  note: ラジエター～大気間
      | 熱抵抗
  note: 冷却水＋ラジエターコア
      | 熱容量
  Temp_ini : Inport
  v_VL_PNT_kmph : Inport  Port=2
  V_ELTH_CNT_RDFan_V : Inport  Port=3
  V_ELTH_CNT_WP_V : Inport  Port=4
  T_ATM_PNT_RD_K : Inport  Port=5
  T_MGTH_PNT_RD_K : Inport  Port=6
  T_INVTH_PNT_RD_K : Inport  Port=7
  Add : Sum
  INV2Coolant_Heat_Resistance1 : Subsystem
  K->degC1 : Subsystem
  MG2Coolant_Heat_Resistance : Subsystem
  RDCoolant2Air_Heat_Resistance : Subsystem
  RDCoolant_Heat_Capacity : Subsystem
  RD_Core_Heat_Resi_Calc : Subsystem
  Water_Pump : Subsystem
  T_RDCoolant_K : Outport
  Heat_Resi_ELTH_PNT_AirconCore_KpW : Outport  Port=2
  PHI_RDTH_PNT_ATM_W : Outport  Port=3
  PHI_RD_PNT_MGTH_W : Outport  Port=4
  PHI_RD_PNT_INVTH_W : Outport  Port=5
  tag scope: tScope_T_RDCoolant_degC=global
  wires:
  RDCoolant_Heat_Capacity/2(T_RDCoolant1_K) -> INV2Coolant_Heat_Resistance1/3(T_Coolant_Resi_K)
  INV2Coolant_Heat_Resistance1/1(PHI_Coolant_Resi_W) -> RDCoolant_Heat_Capacity/2(PHI_RDCoolant1_W)
  RDCoolant2Air_Heat_Resistance/1(PHI_RD_Air_Resi1_W) -> PHI_RDTH_PNT_ATM_W/1
  RDCoolant2Air_Heat_Resistance/2(PHI_RDCoolant_Resi2_W) -> RDCoolant_Heat_Capacity/3(PHI_RDCoolant2_W)
  V_ELTH_CNT_RDFan_V/1 -> RD_Core_Heat_Resi_Calc/1(ELTH_PNT_Voltage_RDFan_V)
  v_VL_PNT_kmph/1 -> RD_Core_Heat_Resi_Calc/2(v_VL_PNT_kmph)
  RD_Core_Heat_Resi_Calc/1("ELTH_PNT_RDCore_Heat_Resi_KpW ") -> RDCoolant2Air_Heat_Resistance/2("RD_PNT_RDCore_Heat_Resi_KpW ")
  T_ATM_PNT_RD_K/1 -> RDCoolant2Air_Heat_Resistance/1(T_RD_Air_Resi1_K)
  RDCoolant_Heat_Capacity/1(T_RDCoolant2_K) -> T_RDCoolant_K/1, K->degC1/1(K), RDCoolant2Air_Heat_Resistance/3(T_RDCoolant_Resi2_K)
  Water_Pump/1(Qv_Coolant_m3ps) -> MG2Coolant_Heat_Resistance/2(Qv_Coolant_m3ps), INV2Coolant_Heat_Resistance1/1(Qv_Coolant_m3ps)
  T_MGTH_PNT_RD_K/1 -> MG2Coolant_Heat_Resistance/3(T_MGTH_Resi2_K)
  MG2Coolant_Heat_Resistance/1(PHI_MGTH_Resi2_W) -> PHI_RD_PNT_MGTH_W/1
  T_INVTH_PNT_RD_K/1 -> MG2Coolant_Heat_Resistance/1(T_Coolant_Resi2_K), INV2Coolant_Heat_Resistance1/2(T_INVTH_Resi_K)
  Add/1 -> PHI_RD_PNT_INVTH_W/1
  INV2Coolant_Heat_Resistance1/2(PHI_INVTH_Resi_W) -> Add/1
  MG2Coolant_Heat_Resistance/2(PHI_Coolant_Resi2_W) -> Add/2
  V_ELTH_CNT_WP_V/1 -> Water_Pump/1(ELTH_PNT_Voltage_WP_V)
  Temp_ini/1 -> RDCoolant_Heat_Capacity/1(Temp_ini)
  RD_Core_Heat_Resi_Calc/2(ELTH_PNT_AirconCore_Heat_Resi_KpW) -> Heat_Resi_ELTH_PNT_AirconCore_KpW/1
  K->degC1/1(degC) -> [tScope_T_RDCoolant_degC]

== system EV_thermal_charger_2015a_20200311/Vehicle/EL_PNT/Divide_0wari1 ==
  In1 : Inport
  In2 : Inport  Port=2
  Constant : Constant  Value=0
  Constant1 : Constant
  Constant2 : Constant  Value=0
  Divide : Product  Inputs=*/
  Logical Operator : Logic  Operator=OR  AllPortsSameDT=off  OutDataTypeStr=boolean
  Relational Operator : RelationalOperator  Operator=>  OutDataTypeStr=boolean
  Relational Operator1 : RelationalOperator  Operator=<  OutDataTypeStr=boolean
  Switch : Switch  Criteria=u2 > Threshold  Threshold=0.5
  Switch1 : Switch  Criteria=u2 > Threshold  Threshold=0.5
  Out1 : Outport
  wires:
  In1/1 -> Divide/1
  Divide/1 -> Switch1/1
  In2/1 -> Relational Operator1/1, Relational Operator/1, Switch/1
  Constant/1 -> Relational Operator1/2, Relational Operator/2
  Relational Operator/1 -> Logical Operator/1
  Relational Operator1/1 -> Logical Operator/2
  Switch/1 -> Divide/2
  Logical Operator/1 -> Switch1/2, Switch/2
  Constant1/1 -> Switch/3
  Constant2/1 -> Switch1/3
  Switch1/1 -> Out1/1

== system EV_thermal_charger_2015a_20200311/Vehicle/EL_PNT/Lo_body_elec_load_resi ==

== system EV_thermal_charger_2015a_20200311/Vehicle/INV_PNT/Divide_0wari1 ==
  ÷ : Inport
  × : Inport  Port=2
  Constant : Constant  Value=0
  Constant1 : Constant
  Constant2 : Constant  Value=0
  Divide : Product  Inputs=*/
  Logical Operator : Logic  Operator=OR  AllPortsSameDT=off  OutDataTypeStr=boolean
  Relational Operator : RelationalOperator  Operator=>  OutDataTypeStr=boolean
  Relational Operator1 : RelationalOperator  Operator=<  OutDataTypeStr=boolean
  Switch : Switch  Criteria=u2 > Threshold  Threshold=0.5
  Switch1 : Switch  Criteria=u2 > Threshold  Threshold=0.5
  "　" : Outport
  wires:
  Switch1/1 -> "　"/1
  Constant2/1 -> Switch1/3
  Constant1/1 -> Switch/3
  Logical Operator/1 -> Switch/2, Switch1/2
  Switch/1 -> Divide/2
  Relational Operator1/1 -> Logical Operator/2
  Relational Operator/1 -> Logical Operator/1
  Constant/1 -> Relational Operator/2, Relational Operator1/2
  ÷/1 -> Switch/1, Relational Operator/1, Relational Operator1/1
  Divide/1 -> Switch1/1
  ×/1 -> Divide/1

== system EV_thermal_charger_2015a_20200311/Vehicle/INV_PNT/Divide_0wari2 ==
  ÷ : Inport
  × : Inport  Port=2
  Constant : Constant  Value=0
  Constant1 : Constant
  Constant2 : Constant  Value=0
  Divide : Product  Inputs=*/
  Logical Operator : Logic  Operator=OR  AllPortsSameDT=off  OutDataTypeStr=boolean
  Relational Operator : RelationalOperator  Operator=>  OutDataTypeStr=boolean
  Relational Operator1 : RelationalOperator  Operator=<  OutDataTypeStr=boolean
  Switch : Switch  Criteria=u2 > Threshold  Threshold=0.5
  Switch1 : Switch  Criteria=u2 > Threshold  Threshold=0.5
  "　" : Outport
  wires:
  Switch1/1 -> "　"/1
  Constant2/1 -> Switch1/3
  Constant1/1 -> Switch/3
  Logical Operator/1 -> Switch/2, Switch1/2
  Switch/1 -> Divide/2
  Relational Operator1/1 -> Logical Operator/2
  Relational Operator/1 -> Logical Operator/1
  Constant/1 -> Relational Operator/2, Relational Operator1/2
  ÷/1 -> Switch/1, Relational Operator/1, Relational Operator1/1
  Divide/1 -> Switch1/1
  ×/1 -> Divide/1

== system EV_thermal_charger_2015a_20200311/Vehicle/INV_PNT/Subsystem ==
  eta : Inport
  OUT_Power : Inport  Port=2
  Constant : Constant
  Product : Product  Inputs=*/
  Product1 : Product
  Saturation : Saturate  UpperLimit=1  LowerLimit=-1
      settings: AttributesFormatString=%<LowerLimit> < u < %<UpperLimit>
  Sum1 : Sum  Inputs=|-+
  Switch : Switch  Criteria=u2 > Threshold
  Loss_Power : Outport
  IN_Power : Outport  Port=2
  wires:
  Sum1/1 -> Loss_Power/1
  Saturation/1 -> Switch/2
  eta/1 -> Switch/3, Product/2
  Constant/1 -> Product/1
  Switch/1 -> Product1/2
  OUT_Power/1 -> Sum1/1, Product1/1, Saturation/1
  Product1/1 -> Sum1/2, IN_Power/1
  Product/1 -> Switch/1

== system EV_thermal_charger_2015a_20200311/Vehicle/MG_CNT/WeakField_Calc ==
  note: u相電圧実効値の最大値
  I_MG_tgt : Inport
  MG_Power_factor : Inport  Port=2
  MG_Mod_factor : Inport  Port=3
  V_INV_PNT_DC_V : Inport  Port=4
  w_MG_PNT_radps : Inport  Port=5
  Abs : Abs
  Constant : Constant  Value=10
  Constant2 : Constant  Value=MG_PNT_MG_WeakField_UL
  Constant3 : Constant  Value=MG_PNT_MG_WeakField_LL
  Divide : Product  Inputs=*/
  Divide1 : Product  Inputs=*/
  MinMax : MinMax  Function=max  Inputs=2
  Product : Product
  Product2 : Product
  Product3 : Product  Inputs=4
  Saturation Dynamic : simulink/Discontinuities/Saturation Dynamic  OutMin=[]  OutMax=[]  OutDataTypeStr=Inherit: Same as second input  OutDataType=fixdt(1, 16)  OutScaling=2^-10  DoSatur=off
  Terminator : Terminator
  定格回転数 : Constant  Value=MG_PNT_w_ROT_MG_Rated
  定格電圧 : Constant  Value=MG_PNT_V_MG_Rated
  線間→u相変換 : Constant  Value=1/sqrt(3)
  k_radps2Volt_tgt : Outport
  wires:
  Divide/1 -> Product/2, Product2/2
  Product2/1 -> k_radps2Volt_tgt/1
  I_MG_tgt/1 -> Terminator/1
  定格電圧/1 -> Divide/1
  定格回転数/1 -> Divide/2
  Product/1 -> Divide1/2
  Product3/1 -> Divide1/1
  線間→u相変換/1 -> Product3/4
  MinMax/1 -> Product/1
  Abs/1 -> MinMax/1
  Constant/1 -> MinMax/2
  w_MG_PNT_radps/1 -> Abs/1
  Saturation Dynamic/1 -> Product2/1
  Divide1/1 -> Saturation Dynamic/2
  Constant2/1 -> Saturation Dynamic/1
  Constant3/1 -> Saturation Dynamic/3
  V_INV_PNT_DC_V/1 -> Product3/3
  MG_Mod_factor/1 -> Product3/2
  MG_Power_factor/1 -> Product3/1

== system EV_thermal_charger_2015a_20200311/Vehicle/MG_CNT/trq_Gurad_Calc ==
  w_MG_PNT_radps : Inport
  Abs : Abs
  Constant : Constant
  Divide1 : Product  Inputs=*/
  Divide2 : Product  Inputs=*/
  Divide_0wari : METI_Lib_vehicle_model/Divide_0wari
  Divide_0wari1 : METI_Lib_vehicle_model/Divide_0wari
  Gain1 : Gain  Gain=-1
  Gain2 : Gain  Gain=-1
  MinMax : MinMax  Inputs=2
  MinMax1 : MinMax  Function=max  Inputs=2
  MinMax2 : MinMax  Function=max  Inputs=2
  Switch : Switch
  Switch1 : Switch
  力行側出力上限 : Constant  Value=MG_CNT_Pmax_MG_Gene_W
  力行側定トルク回転数上限 : Constant  Value=MG_CNT_MG_Const_trq_Gene_radps
  回生側出力上限 : Constant  Value=MG_CNT_Pmin_MG_ReGene_W
  回生側定トルク回転数上限 : Constant  Value=MG_CNT_MG_Const_trq_ReGene_radps
  UpperLimit : Outport
  LowerLimit : Outport  Port=2
  wires:
  w_MG_PNT_radps/1 -> Abs/1, Switch/2, Switch1/2
  MinMax2/1 -> Divide_0wari1/2, Divide_0wari/2
  MinMax1/1 -> Switch1/1, Gain1/1
  MinMax/1 -> Switch/1, Gain2/1
  Gain1/1 -> Switch/3
  Gain2/1 -> Switch1/3
  Switch1/1 -> LowerLimit/1
  Switch/1 -> UpperLimit/1
  力行側定トルク回転数上限/1 -> Divide1/2
  力行側出力上限/1 -> Divide_0wari/1, Divide1/1
  回生側定トルク回転数上限/1 -> Divide2/2
  回生側出力上限/1 -> Divide_0wari1/1, Divide2/1
  Divide1/1 -> MinMax/2
  Divide_0wari/1 -> MinMax/1
  Divide2/1 -> MinMax1/2
  Divide_0wari1/1 -> MinMax1/1
  Abs/1 -> MinMax2/2
  Constant/1 -> MinMax2/1

== system EV_thermal_charger_2015a_20200311/Vehicle/MG_PNT/Power_Conversion ==
  note: U相電流
  note: U-V線間電圧
  note: U相有効電圧
  note: UVW三相合計の
      | モータートルク
  note: U相皮相電圧
  k_MG_CNT_Vpradps : Inport
  Power_factor_INV_PNT : Inport  Port=2
  "w_TM_PNT_radps " : Inport  Port=3
  "I_INV_PNT_AC_A " : Inport  Port=4
  Constant1 : Constant  Value=3
  Constant2 : Constant  Value=sqrt(3)
  Divide : Product  Inputs=/*
  Product{,1,3..4} (4 alike) : Product
  V_MG_PNT_AC_V : Outport
  "trq_Power_Conversion_Nm " : Outport  Port=2
  wires:
  k_MG_CNT_Vpradps/1 -> Product1/1, Product/2
  Product1/1 -> "trq_Power_Conversion_Nm "/1  "trq_UPhase"
  Divide/1 -> Product4/1
  Product3/1 -> Product1/2
  Constant2/1 -> Product4/2
  Constant1/1 -> Product3/1
  "I_INV_PNT_AC_A "/1 -> Product3/2
  Power_factor_INV_PNT/1 -> Divide/1
  Product/1 -> Divide/2
  "w_TM_PNT_radps "/1 -> Product/1
  Product4/1 -> V_MG_PNT_AC_V/1

== system EV_thermal_charger_2015a_20200311/Vehicle/PTTH_PNT/DFTH_PNT ==
  note: T/Mブロックへの熱量
  note: DFオイルの
      | 熱容量
  note: DFブロックの
      | 熱容量
  Temp_ini : Inport
  "T_ATM_PNT_DF_K " : Inport  Port=2
  PHI_DF_PNT_W : Inport  Port=3
  "T_TMTH_PNT_DFTH_K " : Inport  Port=4
  DFBlock2Air_Heat_Resistance : Subsystem
  DFBlock_Heat_Capacity : Subsystem
  DFOil2DFBlock_Heat_Resistance : Subsystem
  DFOil_Heat_Capacity : Subsystem
  K->degC1 : Subsystem
  TMBlock2DFBlock_Heat_Resistance : Subsystem
  "PHI_DFTH_PNT_ATM_W " : Outport
  T_DFTH_PNT_TM_K : Outport  Port=2
  "PHI_DFTH_PNT_TMTH_W " : Outport  Port=3
  tag scope: tScope_T_DFBlock_degC=global
  wires:
  DFOil_Heat_Capacity/2(T_DFOil2_K) -> DFOil2DFBlock_Heat_Resistance/2("T_DFOil_Resi2_K ")
  DFOil2DFBlock_Heat_Resistance/2(PHI_DFOil_Resi2_W) -> DFOil_Heat_Capacity/3("PHI_DFOil2_W ")
  DFOil2DFBlock_Heat_Resistance/1(PHI_DFBlock_Resi1_W) -> DFBlock_Heat_Capacity/2("PHI_DFBlock1_W ")
  DFBlock2Air_Heat_Resistance/2("PHI_DFBlock_Resi3_W ") -> DFBlock_Heat_Capacity/4(PHI_DFBlock3_W)
  DFBlock2Air_Heat_Resistance/1("PHI_DF_Air_Resi1_W ") -> "PHI_DFTH_PNT_ATM_W "/1
  TMBlock2DFBlock_Heat_Resistance/1("PHI_DFBlock_Resi2_W ") -> DFBlock_Heat_Capacity/3("PHI_DFBlock2_W ")
  DFBlock_Heat_Capacity/2(T_DFBlock2_K) -> TMBlock2DFBlock_Heat_Resistance/1("T_DFBlock_Resi2_K ")
  "T_TMTH_PNT_DFTH_K "/1 -> TMBlock2DFBlock_Heat_Resistance/2("T_TMBlock_Resi4_K ")
  TMBlock2DFBlock_Heat_Resistance/2("PHI_TMBlock_Resi4_W ") -> "PHI_DFTH_PNT_TMTH_W "/1
  PHI_DF_PNT_W/1 -> DFOil_Heat_Capacity/2(PHI_DFOil1_W)
  Temp_ini/1 -> DFBlock_Heat_Capacity/1(Temp_ini), DFOil_Heat_Capacity/1(Temp_ini)
  K->degC1/1(degC) -> [tScope_T_DFBlock_degC]
  "T_ATM_PNT_DF_K "/1 -> DFBlock2Air_Heat_Resistance/2(T_DF_Air_Resi1_K)
  DFBlock_Heat_Capacity/3("T_DFBlock3_K ") -> DFBlock2Air_Heat_Resistance/1("T_DFBlock_Resi3_K "), K->degC1/1(K)
  DFBlock_Heat_Capacity/1("T_DFBlock1_K ") -> DFOil2DFBlock_Heat_Resistance/1(T_DFBlock_Resi1_K)
  DFOil_Heat_Capacity/1("T_DFOil1_K ") -> T_DFTH_PNT_TM_K/1

== system EV_thermal_charger_2015a_20200311/Vehicle/PTTH_PNT/K->degC6 ==
  K : Inport
  Constant2 : Constant  Value=K2degC
  Sum : Sum  Inputs=++|
  degC : Outport
  wires:
  K/1 -> Sum/2
  Constant2/1 -> Sum/1
  Sum/1 -> degC/1

== system EV_thermal_charger_2015a_20200311/Vehicle/PTTH_PNT/TMTH_PNT ==
  note: TFの
      | 熱容量
  note: T/Mブロックの
      | 熱容量
  note: DFブロックからの熱量
  note: TMからの熱量
  note: T/Mブロックから大気へ
      | 放熱する熱量
  note: モーターハウジングからの熱量
  Temp_ini : Inport
  PHI_TM_PNT_W : Inport  Port=2
  "PHI_MGTH_PNT_PTTH_W " : Inport  Port=3
  "T_ATM_PNT_TM_K " : Inport  Port=4
  "PHI_DFTH_PNT_TMTH_W " : Inport  Port=5
  K->degC1 : Subsystem
  TF2TMBlock_Heat_Resistance : Subsystem
  TF_Heat_Capacity : Subsystem
  TMBlock2Air_Heat_Resistance : Subsystem
  TMBlock_Heat_Capacity : Subsystem
  T_TMTH_PNT_DFTH_K : Outport
  PHI_TMTH_PNT_ATM_W : Outport  Port=2
  T_TMTH_PNT_ELTH_K : Outport  Port=3
  "T_TMTH_PNT_TM_K " : Outport  Port=4
  T_TF_K : Outport  Port=5
  tag scope: tScope_T_TMBlock_degC=global
  wires:
  TF_Heat_Capacity/2(T_TF2_K) -> TF2TMBlock_Heat_Resistance/2("T_TF_Resi2_K ")
  TF2TMBlock_Heat_Resistance/2(PHI_TF_Resi2_W) -> TF_Heat_Capacity/3(PHI_TF2_W)
  TMBlock_Heat_Capacity/1(T_TMBlock1_K) -> TF2TMBlock_Heat_Resistance/1("T_TMBlock_Resi1_K ")
  TF2TMBlock_Heat_Resistance/1(PHI_TMBlock_Resi1_W) -> TMBlock_Heat_Capacity/2(PHI_TMBlock1_W)
  TF_Heat_Capacity/1(T_TF1_K) -> T_TF_K/1, "T_TMTH_PNT_TM_K "/1
  TMBlock2Air_Heat_Resistance/2(PHI_TMBlock_Resi3_W) -> TMBlock_Heat_Capacity/3(PHI_TMBlock2_W)
  TMBlock_Heat_Capacity/2(T_TMBlock2_K) -> TMBlock2Air_Heat_Resistance/2("T_TMBlock_Resi3_K ")
  TMBlock_Heat_Capacity/3(T_TMBlock3_K) -> T_TMTH_PNT_DFTH_K/1
  "PHI_DFTH_PNT_TMTH_W "/1 -> TMBlock_Heat_Capacity/4(PHI_TMBlock3_W)
  "T_ATM_PNT_TM_K "/1 -> TMBlock2Air_Heat_Resistance/1(T_TM_Air_Resi1_K)
  TMBlock2Air_Heat_Resistance/1("PHI_TM_Air_Resi1_W ") -> PHI_TMTH_PNT_ATM_W/1
  TMBlock_Heat_Capacity/4(T_TMBlock4_K) -> K->degC1/1(K), T_TMTH_PNT_ELTH_K/1
  Temp_ini/1 -> TMBlock_Heat_Capacity/1(Temp_ini), TF_Heat_Capacity/1(Temp_ini)
  K->degC1/1(degC) -> [tScope_T_TMBlock_degC]
  "PHI_MGTH_PNT_PTTH_W "/1 -> TMBlock_Heat_Capacity/5(PHI_TMBlock4_W)
  PHI_TM_PNT_W/1 -> TF_Heat_Capacity/2(PHI_TF1_W)

== system EV_thermal_charger_2015a_20200311/Vehicle/TM_PNT/Flywheel1 ==
  Trq_DF_PNT_UP_Nm : Inport
  Trq_TM_Flywheel_UP : Inport  Port=2
  Discrete-Time Integrator : DiscreteIntegrator  InitialConditionSetting=State (most efficient)  SampleTime=sampling_time  LowerSaturationLimit=0
  Divide : Product  Inputs=/*
  Inertia : Constant  Value=TM_PNT_TM_Inertia
  Sum : Sum  Inputs=++|
  w_TM_PNT_DN_radps : Outport
  "w_ROT_TM_Flywheel_UP " : Outport  Port=2
  wires:
  Trq_DF_PNT_UP_Nm/1 -> Sum/1
  Sum/1 -> Divide/2
  Inertia/1 -> Divide/1
  Divide/1 -> Discrete-Time Integrator/1
  Discrete-Time Integrator/1 -> w_TM_PNT_DN_radps/1, "w_ROT_TM_Flywheel_UP "/1
  Trq_TM_Flywheel_UP/1 -> Sum/2
